simulink model "HIL_model_experiments1"  (R2013a)
settings: Solver=ode5  StartTime=0.0  StopTime=simulationTime  FixedStep=0.1  RelTol=1e-3
values from neighbouring files (symbols this model uses):
  Di = [50 0 ... (first row only)    [theProgram.m]
  Dist_spv_rfp = sqrt( ( shipL_d(1) - Rfp(1) )^2 + (shipL_d(2) - Rfp(2) )^2 )    [theProgram.m]
  Ds = [-X_u 0 0 ... (first row only)    [theProgram.m]
  K_M = [ 1 0 0 ... (first row only)    [theProgram.m]
  K_tow = 20    [theProgram.m]
  kappa = 2    [theProgram.m]
  Mi_a = iceMass*[1 0; 0 1]    [theProgram.m]
  Mi_rb = iceMass*[1 0; 0 1]    [theProgram.m]
  Ms_a = -[X_udot 0 0 ... (first row only)    [theProgram.m]
  Ms_rb = [shipMass 0 0 ... (first row only)    [theProgram.m]
  Ninstances = 50    [theProgram.m]
  overturnLimit = 4    [theProgram.m]
  Piceberg = [-4.5; -2.9]    [theProgram.m]
  Pship = [-3.5; -2.9; 0]    [theProgram.m]
  ruptureLimit = 3    [theProgram.m]
  saved_init = zeros(Ninstances,1)    [theProgram.m]
  sd_break = 0.075*T_break    (= 12)    [theProgram.m]
  sd_overturn = 0.075*T_overturn    (= 9.75)    [theProgram.m]
  sd_slip = 0.075*T_slip    (= 10.5)    [theProgram.m]
  simCase = 1    [theProgram.m]
  slippageLimit = 5    [theProgram.m]
  T_break = 160    [theProgram.m]
  T_overturn = 130    [theProgram.m]
  T_slip = 140    [theProgram.m]
  TowLineLength = 1.11    [theProgram.m]
  Vc = [cVelocity*cos(cAngle) ... (first row only)    [theProgram.m]
  vesselForces = [4; -1; 0]    [theProgram.m]
libraries: dspmtrx3 x1
settings Model: Creator=Andreas  LastModifiedBy=Andreas

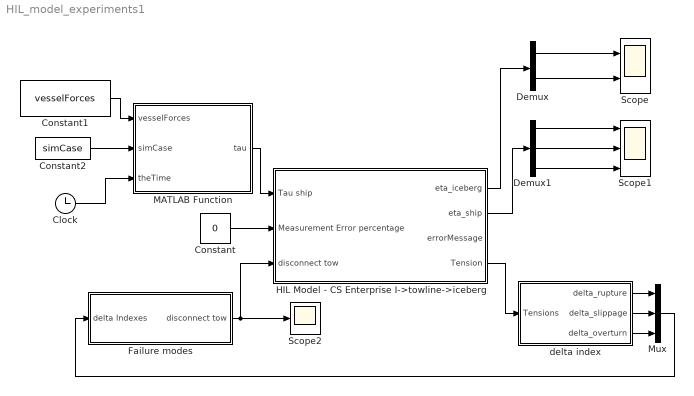
== system HIL_model_experiments1 ==
  Clock : Clock
  Constant : Constant  Value=0
  Constant1 : Constant  Value=vesselForces  VectorParams1D=off
  Constant2 : Constant  Value=simCase
  Demux : Demux  Outputs=2
  Demux1 : Demux  Outputs=3
  Failure modes : Subsystem
  HIL Model - CS Enterprise I->towline->iceberg : Subsystem  VariantControl=Variant1
  MATLAB Function : MATLAB Function  TreatAsAtomicUnit=on
  Mux : Mux  Inputs=3
  Scope : Scope  NumInputPorts=2
      settings: YMin=-5~-5  YMax=5~5  SaveName=ScopeData5
  Scope1 : Scope  NumInputPorts=3
      settings: YMin=-5~-5~-5  YMax=5~5~5  SaveName=ScopeData6
  Scope2 : Scope
      settings: SaveName=ScopeData7
  delta index : Subsystem
  wires:
  Constant/1 -> HIL Model - CS Enterprise I->towline->iceberg/2(Measurement Error percentage)
  HIL Model - CS Enterprise I->towline->iceberg/4(Tension) -> delta index/1(Tensions)
  Failure modes/1(disconnect tow) -> HIL Model - CS Enterprise I->towline->iceberg/3(disconnect tow), Scope2/1
  delta index/2(delta_slippage) -> Mux/2
  delta index/3(delta_overturn) -> Mux/3
  delta index/1(delta_rupture) -> Mux/1
  Mux/1 -> Failure modes/1(delta Indexes)
  HIL Model - CS Enterprise I->towline->iceberg/1(eta_iceberg) -> Demux/1
  Demux/2 -> Scope/2
  Demux/1 -> Scope/1
  HIL Model - CS Enterprise I->towline->iceberg/2(eta_ship) -> Demux1/1
  Demux1/2 -> Scope1/2
  Demux1/3 -> Scope1/3
  Demux1/1 -> Scope1/1
  MATLAB Function/1(tau) -> HIL Model - CS Enterprise I->towline->iceberg/1(Tau ship)
  Constant1/1 -> MATLAB Function/1(vesselForces)
  Constant2/1 -> MATLAB Function/2(simCase)
  Clock/1 -> MATLAB Function/3(theTime)

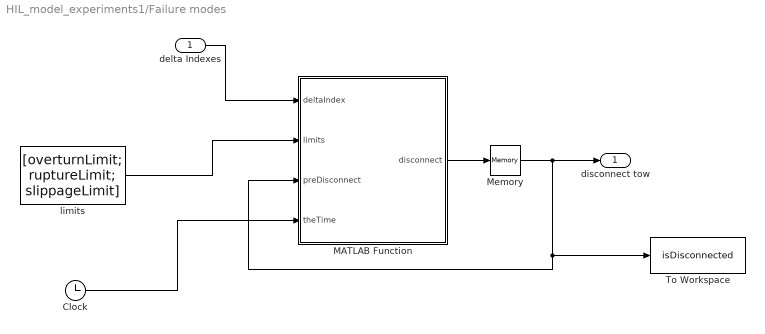
== system HIL_model_experiments1/Failure modes ==
  delta Indexes : Inport
  Clock : Clock
  MATLAB Function : MATLAB Function  TreatAsAtomicUnit=on
  Memory : Memory
  To Workspace : ToWorkspace  VariableName=isDisconnected  SampleTime=-1  SaveFormat=Timeseries
  limits : Constant  Value=[overturnLimit; ruptureLimit; slippageLimit]  VectorParams1D=off
  disconnect tow : Outport
  wires:
  limits/1 -> MATLAB Function/2(limits)
  delta Indexes/1 -> MATLAB Function/1(deltaIndex)
  Clock/1 -> MATLAB Function/4(theTime)
  MATLAB Function/1(disconnect) -> Memory/1
  Memory/1 -> MATLAB Function/3(preDisconnect), To Workspace/1, disconnect tow/1

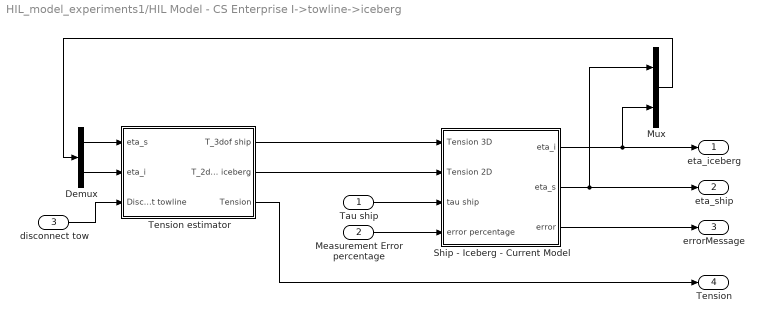
== system HIL_model_experiments1/HIL Model - CS Enterprise I->towline->iceberg ==
  Tau ship : Inport
  Measurement Error percentage : Inport  Port=2
  disconnect tow : Inport  Port=3
  Demux : Demux  Outputs=2
  Mux : Mux  Inputs=[3; 2]
  Ship - Iceberg - Current Model : Subsystem
  Tension estimator : Subsystem
  eta_iceberg : Outport
  eta_ship : Outport  Port=2
  errorMessage : Outport  Port=3
  Tension : Outport  Port=4
  wires:
  Tension estimator/2(T_2dof iceberg) -> Ship - Iceberg - Current Model/2(Tension 2D)
  Tension estimator/1(T_3dof ship) -> Ship - Iceberg - Current Model/1(Tension 3D)
  Measurement Error percentage/1 -> Ship - Iceberg - Current Model/4(error percentage)
  Demux/2 -> Tension estimator/2(eta_i)
  Ship - Iceberg - Current Model/1(eta_i) -> Mux/2, eta_iceberg/1
  Demux/1 -> Tension estimator/1(eta_s)
  Tau ship/1 -> Ship - Iceberg - Current Model/3(tau ship)
  Ship - Iceberg - Current Model/3(error) -> errorMessage/1
  Mux/1 -> Demux/1
  Ship - Iceberg - Current Model/2(eta_s) -> Mux/1, eta_ship/1
  Tension estimator/3(Tension) -> Tension/1
  disconnect tow/1 -> Tension estimator/3(Disconnect towline)

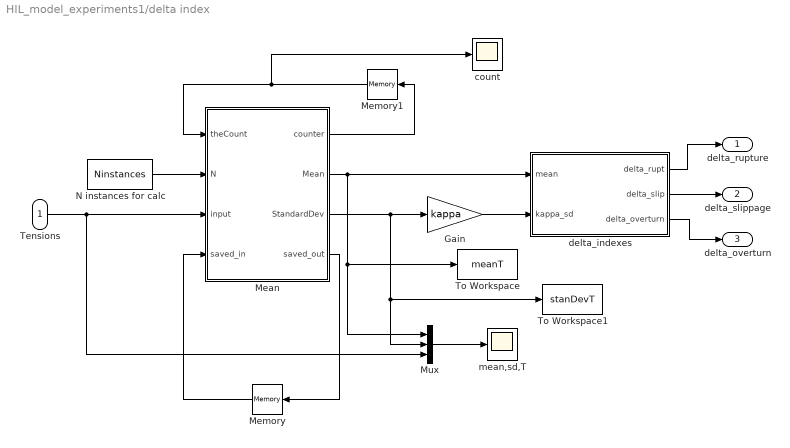
== system HIL_model_experiments1/delta index ==
  Tensions : Inport
  Gain : Gain  Gain=kappa
  Mean : MATLAB Function  TreatAsAtomicUnit=on
  Memory : Memory  X0=saved_init
  Memory1 : Memory  X0=1
  Mux : Mux  Inputs=3
  N instances for calc : Constant  Value=Ninstances
  To Workspace : ToWorkspace  VariableName=meanT  SampleTime=-1  SaveFormat=Timeseries
  To Workspace1 : ToWorkspace  VariableName=stanDevT  SampleTime=-1  SaveFormat=Timeseries
  count : Scope
  delta_indexes : Subsystem
  mean,sd,T : Scope
      settings: SaveName=ScopeData2
  delta_rupture : Outport
  delta_slippage : Outport  Port=2
  delta_overturn : Outport  Port=3
  wires:
  Mux/1 -> mean,sd,T/1
  Memory/1 -> Mean/4(saved_in)
  Memory1/1 -> Mean/1(theCount), count/1
  Mean/3(StandardDev) -> To Workspace1/1, Mux/2, Gain/1
  Mean/1(counter) -> Memory1/1
  N instances for calc/1 -> Mean/2(N)
  Mean/4(saved_out) -> Memory/1
  Mean/2(Mean) -> Mux/1, To Workspace/1, delta_indexes/1(mean)
  Tensions/1 -> Mux/3, Mean/3(input)
  Gain/1 -> delta_indexes/2(kappa_sd)
  delta_indexes/1(delta_rupt) -> delta_rupture/1
  delta_indexes/2(delta_slip) -> delta_slippage/1
  delta_indexes/3(delta_overturn) -> delta_overturn/1

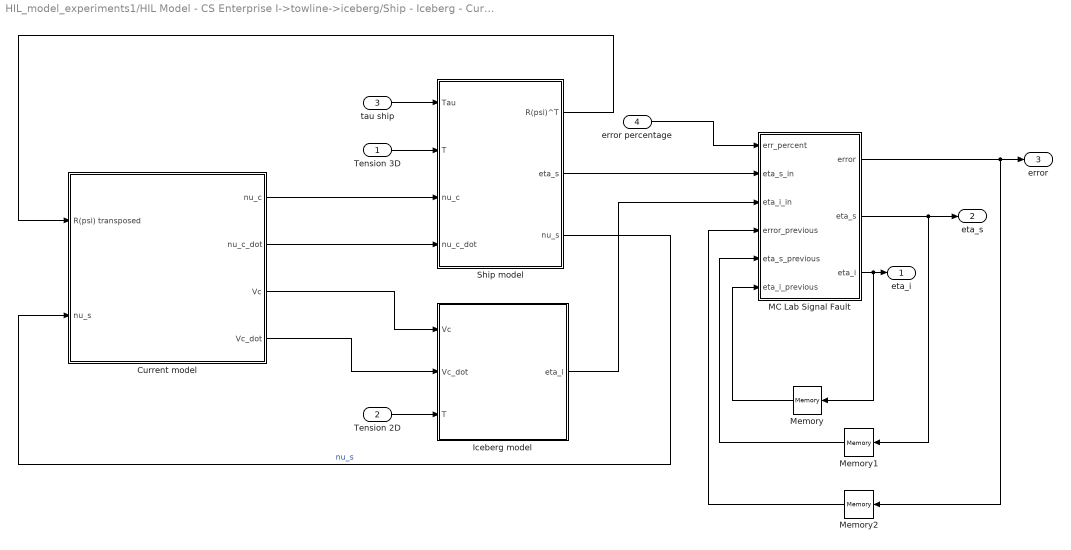
== system HIL_model_experiments1/HIL Model - CS Enterprise I->towline->iceberg/Ship - Iceberg - Current Model ==
  Tension 3D : Inport
  Tension 2D : Inport  Port=2
  tau ship : Inport  Port=3
  error percentage : Inport  Port=4
  Current model : Subsystem
  Iceberg model : Subsystem
  MC Lab Signal Fault : MATLAB Function  TreatAsAtomicUnit=on
  Memory : Memory  X0=[0; 0]
  Memory1 : Memory  X0=[0; 0; 0]
  Memory2 : Memory
  Ship model : Subsystem
  eta_i : Outport
  eta_s : Outport  Port=2
  error : Outport  Port=3
  wires:
  Memory2/1 -> MC Lab Signal Fault/4(error_previous)
  Memory1/1 -> MC Lab Signal Fault/5(eta_s_previous)
  Memory/1 -> MC Lab Signal Fault/6(eta_i_previous)
  MC Lab Signal Fault/1(error) -> error/1, Memory2/1
  MC Lab Signal Fault/3(eta_i) -> eta_i/1, Memory/1
  MC Lab Signal Fault/2(eta_s) -> eta_s/1, Memory1/1
  Iceberg model/1(eta_i) -> MC Lab Signal Fault/3(eta_i_in)
  Ship model/2(eta_s) -> MC Lab Signal Fault/2(eta_s_in)
  error percentage/1 -> MC Lab Signal Fault/1(err_percent)
  Ship model/3(nu_s) -> Current model/2(nu_s)  "nu_s"
  Ship model/1(R(psi)^T) -> Current model/1(R(psi) transposed)
  Tension 2D/1 -> Iceberg model/3(T)
  Current model/4(Vc_dot) -> Iceberg model/2(Vc_dot)
  Current model/3(Vc) -> Iceberg model/1(Vc)
  Current model/2(nu_c_dot) -> Ship model/4(nu_c_dot)
  Current model/1(nu_c) -> Ship model/3(nu_c)
  Tension 3D/1 -> Ship model/2(T)
  tau ship/1 -> Ship model/1(Tau)

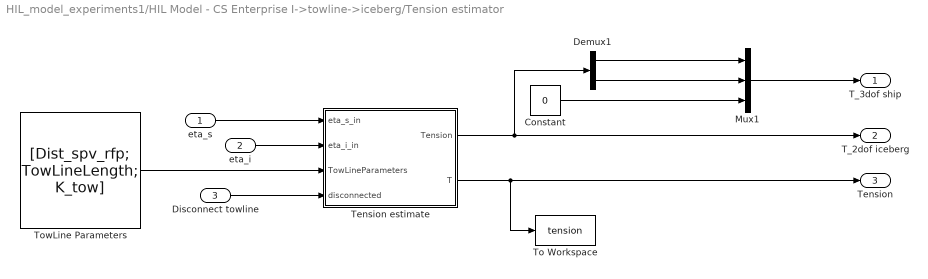
== system HIL_model_experiments1/HIL Model - CS Enterprise I->towline->iceberg/Tension estimator ==
  eta_s : Inport
  eta_i : Inport  Port=2
  Disconnect towline : Inport  Port=3
  Constant : Constant  Value=0
  Demux1 : Demux  Outputs=2
  Mux1 : Mux  Inputs=3
  Tension estimate : MATLAB Function  TreatAsAtomicUnit=on
  To Workspace : ToWorkspace  VariableName=tension  SampleTime=-1  SaveFormat=Timeseries
  TowLine Parameters : Constant  Value=[Dist_spv_rfp; TowLineLength; K_tow]  VectorParams1D=off
  T_3dof ship : Outport
  T_2dof iceberg : Outport  Port=2
  Tension : Outport  Port=3
  wires:
  Tension estimate/1(Tension) -> T_2dof iceberg/1, Demux1/1
  TowLine Parameters/1 -> Tension estimate/3(TowLineParameters)
  Constant/1 -> Mux1/3
  Demux1/2 -> Mux1/2
  Demux1/1 -> Mux1/1
  Mux1/1 -> T_3dof ship/1
  eta_s/1 -> Tension estimate/1(eta_s_in)
  eta_i/1 -> Tension estimate/2(eta_i_in)
  Tension estimate/2(T) -> To Workspace/1, Tension/1
  Disconnect towline/1 -> Tension estimate/4(disconnected)

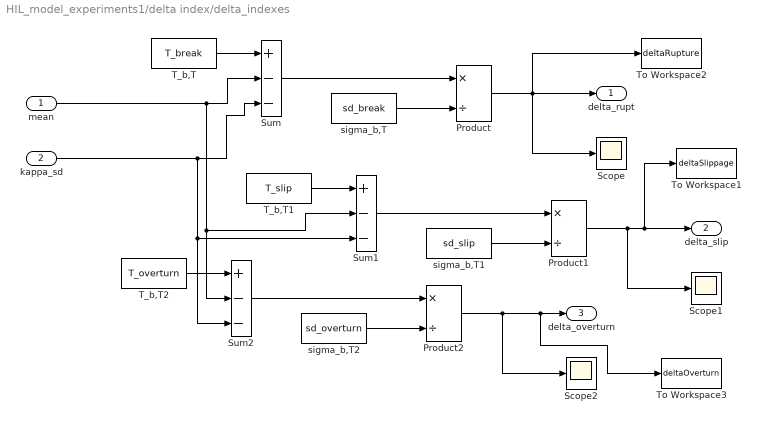
== system HIL_model_experiments1/delta index/delta_indexes ==
  mean : Inport
  kappa_sd : Inport  Port=2
  Product : Product  Inputs=*/
  Product1 : Product  Inputs=*/
  Product2 : Product  Inputs=*/
  Scope : Scope
  Scope1 : Scope
      settings: SaveName=ScopeData3
  Scope2 : Scope
      settings: SaveName=ScopeData4
  Sum : Sum  Inputs=+--
  Sum1 : Sum  Inputs=+--
  Sum2 : Sum  Inputs=+--
  T_b,T : Constant  Value=T_break
  T_b,T1 : Constant  Value=T_slip
  T_b,T2 : Constant  Value=T_overturn
  To Workspace1 : ToWorkspace  VariableName=deltaSlippage  SampleTime=-1  SaveFormat=Timeseries
  To Workspace2 : ToWorkspace  VariableName=deltaRupture  SampleTime=-1  SaveFormat=Timeseries
  To Workspace3 : ToWorkspace  VariableName=deltaOverturn  SampleTime=-1  SaveFormat=Timeseries
  sigma_b,T : Constant  Value=sd_break
  sigma_b,T1 : Constant  Value=sd_slip
  sigma_b,T2 : Constant  Value=sd_overturn
  delta_rupt : Outport
  delta_slip : Outport  Port=2
  delta_overturn : Outport  Port=3
  wires:
  Product/1 -> To Workspace2/1, delta_rupt/1, Scope/1
  kappa_sd/1 -> Sum2/3, Sum1/3, Sum/3
  sigma_b,T/1 -> Product/2
  Sum/1 -> Product/1
  T_b,T/1 -> Sum/1
  mean/1 -> Sum2/2, Sum1/2, Sum/2
  Product1/1 -> To Workspace1/1, delta_slip/1, Scope1/1
  sigma_b,T1/1 -> Product1/2
  Sum1/1 -> Product1/1
  T_b,T1/1 -> Sum1/1
  Product2/1 -> To Workspace3/1, delta_overturn/1, Scope2/1
  sigma_b,T2/1 -> Product2/2
  Sum2/1 -> Product2/1
  T_b,T2/1 -> Sum2/1

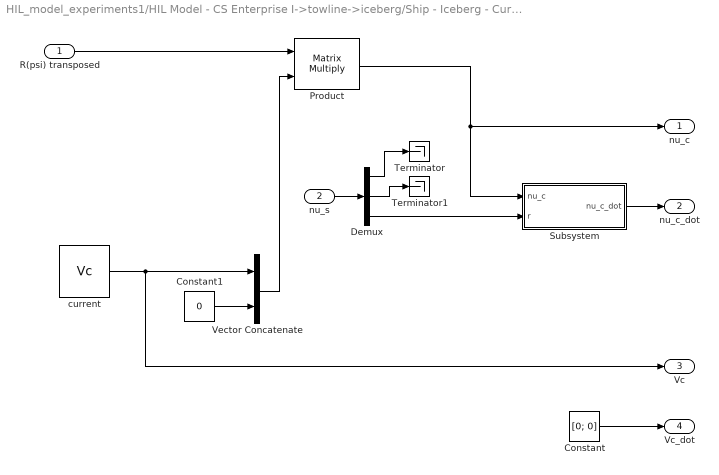
== system HIL_model_experiments1/HIL Model - CS Enterprise I->towline->iceberg/Ship - Iceberg - Current Model/Current model ==
  R(psi) transposed : Inport
  nu_s : Inport  Port=2
  Constant : Constant  Value=[0; 0]  VectorParams1D=off
  Constant1 : Constant  Value=0
  Demux : Demux  Outputs=3
  Product : Product  Multiplication=Matrix(*)
  Subsystem : Subsystem
  Terminator : Terminator
  Terminator1 : Terminator
  Vector Concatenate : Concatenate  Mode=Multidimensional array
  current : Constant  Value=Vc  VectorParams1D=off
  nu_c : Outport
  nu_c_dot : Outport  Port=2
  Vc : Outport  Port=3
  Vc_dot : Outport  Port=4
  wires:
  Vector Concatenate/1 -> Product/2
  Constant1/1 -> Vector Concatenate/2
  Constant/1 -> Vc_dot/1
  Subsystem/1(nu_c_dot) -> nu_c_dot/1
  Demux/3 -> Subsystem/2(r)
  Demux/2 -> Terminator1/1
  Demux/1 -> Terminator/1
  nu_s/1 -> Demux/1
  Product/1 -> nu_c/1, Subsystem/1(nu_c)
  R(psi) transposed/1 -> Product/1
  current/1 -> Vector Concatenate/1, Vc/1

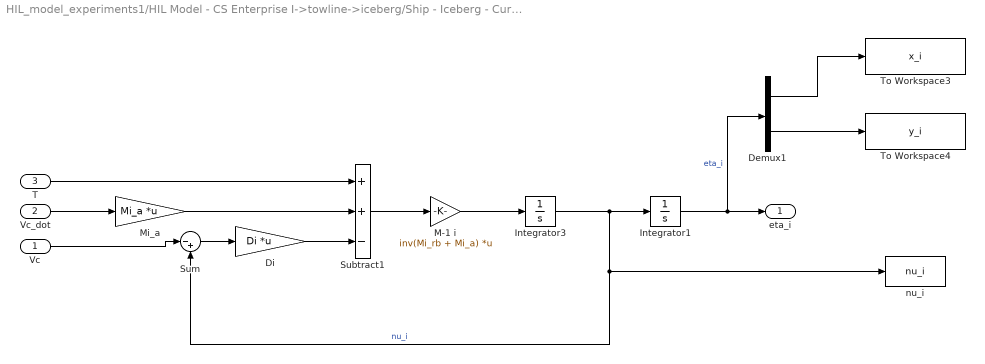
== system HIL_model_experiments1/HIL Model - CS Enterprise I->towline->iceberg/Ship - Iceberg - Current Model/Iceberg model ==
  Vc : Inport
  Vc_dot : Inport  Port=2
  T : Inport  Port=3
  Demux1 : Demux  Outputs=2
  Di : Gain  Gain=Di  Multiplication=Matrix(K*u) (u vector)
  Integrator1 : Integrator  InitialCondition=Piceberg
  Integrator3 : Integrator  InitialCondition=[0;0]
  M-1 i : Gain  Gain=inv(Mi_rb + Mi_a)  Multiplication=Matrix(K*u)
  Mi_a : Gain  Gain=Mi_a  Multiplication=Matrix(K*u) (u vector)
  Subtract1 : Sum  Inputs=++-
  Sum : Sum  Inputs=|-+
  To Workspace3 : ToWorkspace  VariableName=x_i  SampleTime=-1  SaveFormat=Timeseries
  To Workspace4 : ToWorkspace  VariableName=y_i  SampleTime=-1  SaveFormat=Timeseries
  nu_i : ToWorkspace  VariableName=nu_i  SampleTime=-1  SaveFormat=Timeseries
  eta_i : Outport
  wires:
  Demux1/2 -> To Workspace4/1
  Demux1/1 -> To Workspace3/1
  Di/1 -> Subtract1/3
  Sum/1 -> Di/1
  Vc/1 -> Sum/1
  Mi_a/1 -> Subtract1/2
  Vc_dot/1 -> Mi_a/1
  T/1 -> Subtract1/1
  Subtract1/1 -> M-1 i/1
  M-1 i/1 -> Integrator3/1
  Integrator1/1 -> eta_i/1, Demux1/1  "eta_i"
  Integrator3/1 -> Integrator1/1, nu_i/1, Sum/2  "nu_i"

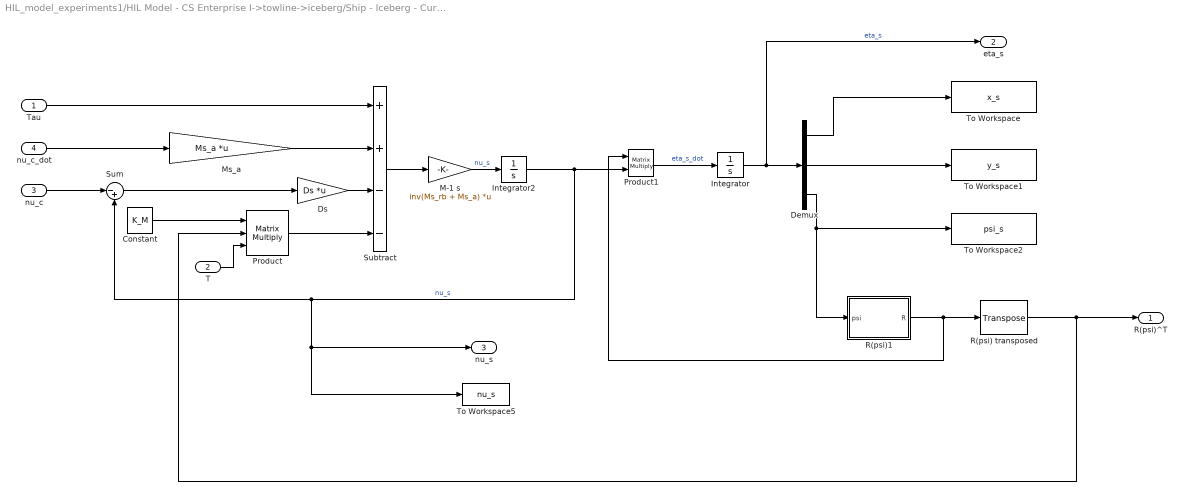
== system HIL_model_experiments1/HIL Model - CS Enterprise I->towline->iceberg/Ship - Iceberg - Current Model/Ship model ==
  Tau : Inport
  T : Inport  Port=2
  nu_c : Inport  Port=3
  nu_c_dot : Inport  Port=4
  Constant : Constant  Value=K_M  VectorParams1D=off
  Demux : Demux  Outputs=3
  Ds : Gain  Gain=Ds  Multiplication=Matrix(K*u) (u vector)
  Integrator : Integrator  InitialCondition=Pship
  Integrator2 : Integrator  InitialCondition=[0; 0; 0]
  M-1 s : Gain  Gain=inv(Ms_rb + Ms_a)  Multiplication=Matrix(K*u) (u vector)
  Ms_a : Gain  Gain=Ms_a  Multiplication=Matrix(K*u) (u vector)
  Product : Product  Inputs=***  Multiplication=Matrix(*)
  Product1 : Product  Multiplication=Matrix(*)
  R(psi) transposed : dspmtrx3/Transpose  Hermitian=off  overflowFlag=off
  R(psi)1 : MATLAB Function  TreatAsAtomicUnit=on
  Subtract : Sum  Inputs=++--
  Sum : Sum  Inputs=|-+
  To Workspace : ToWorkspace  VariableName=x_s  SampleTime=-1  SaveFormat=Timeseries
  To Workspace1 : ToWorkspace  VariableName=y_s  SampleTime=-1  SaveFormat=Timeseries
  To Workspace2 : ToWorkspace  VariableName=psi_s  SampleTime=-1  SaveFormat=Timeseries
  To Workspace5 : ToWorkspace  VariableName=nu_s  SampleTime=-1  SaveFormat=Timeseries
  R(psi)^T : Outport
  eta_s : Outport  Port=2
  nu_s : Outport  Port=3
  wires:
  Tau/1 -> Subtract/1
  R(psi) transposed/1 -> Product/2, R(psi)^T/1
  Demux/3 -> To Workspace2/1, R(psi)1/1(psi)
  Demux/2 -> To Workspace1/1
  Demux/1 -> To Workspace/1
  Product1/1 -> Integrator/1  "eta_s_dot"
  R(psi)1/1(R) -> Product1/1, R(psi) transposed/1
  Constant/1 -> Product/1
  Subtract/1 -> M-1 s/1
  M-1 s/1 -> Integrator2/1  "nu_s"
  Ds/1 -> Subtract/3
  Ms_a/1 -> Subtract/2
  Integrator/1 -> Demux/1, eta_s/1  "eta_s"
  T/1 -> Product/3
  nu_c/1 -> Sum/1
  Sum/1 -> Ds/1
  Integrator2/1 -> Product1/2, nu_s/1, To Workspace5/1, Sum/2  "nu_s"
  Product/1 -> Subtract/4
  nu_c_dot/1 -> Ms_a/1

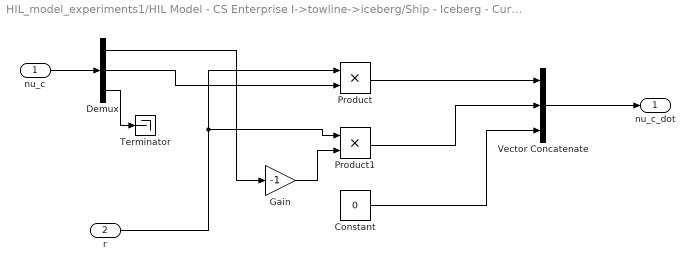
== system HIL_model_experiments1/HIL Model - CS Enterprise I->towline->iceberg/Ship - Iceberg - Current Model/Current model/Subsystem ==
  nu_c : Inport
  r : Inport  Port=2
  Constant : Constant  Value=0
  Demux : Demux  Outputs=3
  Gain : Gain  Gain=-1
  Product : Product
  Product1 : Product
  Terminator : Terminator
  Vector Concatenate : Concatenate  NumInputs=3  Mode=Multidimensional array
  nu_c_dot : Outport
  wires:
  Gain/1 -> Product1/2
  Demux/1 -> Gain/1
  Demux/2 -> Product/2
  r/1 -> Product/1, Product1/1
  Constant/1 -> Vector Concatenate/3
  Product1/1 -> Vector Concatenate/2
  Product/1 -> Vector Concatenate/1
  Vector Concatenate/1 -> nu_c_dot/1
  Demux/3 -> Terminator/1
  nu_c/1 -> Demux/1

== matlab function HIL_model_experiments1/HIL Model - CS Enterprise I->towline->iceberg/Ship - Iceberg - Current Model/MC Lab Signal Fault ==
  data: error output; err_percent input; eta_s output; eta_s_in input; eta_i_in input; error_previous input; eta_s_previous input; eta_i_previous input; eta_i output
function [error, eta_s, eta_i] = fcn(err_percent, eta_s_in, eta_i_in, error_previous, eta_s_previous, eta_i_previous)
%#codegen


% Random number generator 0-100
num = 100*rand;

if error_previous == 1
    err_percent = 95;
end

% Check if the num is below the error percentage
if num < err_percent
    error = 1;
    eta_s = eta_s_previous;
    eta_i = eta_i_previous;
else
    error = 0;
    eta_s = eta_s_in;
    eta_i = eta_i_in;
end

== matlab function HIL_model_experiments1/HIL Model - CS Enterprise I->towline->iceberg/Ship - Iceberg - Current Model/Ship model/R(psi)1 ==
  data: psi input; R output
function R = fcn(psi)

c = cos(psi);
s = sin(psi);

R = [c -s 0;
     s c 0;
     0 0 1];

== matlab function HIL_model_experiments1/delta index/Mean ==
  data: counter output; theCount input; N input; Mean output; StandardDev output; input input; saved_in input; saved_out output
function [counter, Mean, StandardDev, saved_out] = fcn(theCount, N, input, saved_in)
%#codegen

meanSum = 0;
varSum = 0;

N = round(N);

startval = 2;
Ndiv = N;
if theCount < N
    startval = N + 1 - theCount;
    Ndiv = theCount;
end

% Bump all saved instances up
saved_out = saved_in;
for i=startval:N
    saved_out(i-1) = saved_in(i);
    meanSum = meanSum + saved_in(i);
end
saved_out(N) = input;
meanSum = meanSum + input;

Mean = (1/Ndiv)*meanSum;


% Calculate variance sum
for i=startval-1:N
    varSum = (saved_out(i) - Mean)^2;
end

variance = (1/Ndiv)*varSum;
StandardDev = sqrt(variance);

counter = theCount + 1;

== matlab function HIL_model_experiments1/HIL Model - CS Enterprise I->towline->iceberg/Tension estimator/Tension estimate ==
  data: eta_s_in input; Tension output; eta_i_in input; TowLineParameters input; T output; disconnected input
function [Tension, T] = fcn(eta_s_in,eta_i_in,TowLineParameters, disconnected)
%#codegen

if length(eta_s_in) > 1
    eta_s = eta_s_in;
else
    eta_s = [0; 0; 0];
end
if length(eta_i_in) > 1
    eta_i = eta_i_in;
else
    eta_i = [0; 0];
end

if disconnected == 0

    d = TowLineParameters(1);
    Tlength = TowLineParameters(2);
    K_tow = TowLineParameters(3);

    x_s = eta_s(1);
    y_s = eta_s(2);
    psi_s = eta_s(3);

    x_i = eta_i(1);
    y_i = eta_i(2);

    % Find rope fastening position in cartesian
    x_r = x_s - d*cos(psi_s);
    y_r = y_s - d*sin(psi_s);

    % Find towline fastening distance and angle
    dist = sqrt( (x_r - x_i)^2 + (y_r - y_i)^2 );
    angle = atan2(y_r-y_i, x_r-x_i);

    % Check if longer than rope length, because only rope stretching tension gives force
    T = 0;
    if dist >= Tlength

        deltaL = dist-Tlength;
        T = K_tow*deltaL;

    end

    % Make Xtow and Ytow
    Xtow = T*cos(angle);
    Ytow = T*sin(angle);

    Tension = [Xtow; Ytow];

else
    
    T = 0;
    Tension = [0; 0];
    
end

== matlab function HIL_model_experiments1/Failure modes/MATLAB Function ==
  data: deltaIndex input; disconnect output; limits input; preDisconnect input; theTime input
function disconnect = fcn(deltaIndex, limits, preDisconnect, theTime)
%#codegen

disconnect = preDisconnect;

if preDisconnect == 0 && theTime > 0

    deltaOverturn = deltaIndex(3);
    deltaRupture = deltaIndex(1);
    deltaSlippage = deltaIndex(2);
    
    overturn = limits(1);
    rupture = limits(2);
    slippage = limits(3);
    
    if deltaOverturn < overturn

        theTime
        disp('Iceberg has overturned, towline is disconnected.');
        disconnect = 1;
        
    elseif deltaRupture < rupture
        
        theTime
        disp('Towline has ruptured, and is disconnected.');
        disconnect = 1;
        
    elseif deltaSlippage < slippage
        
        theTime
        disp('Towline has slipped, and is disconnected.');
        disconnect = 1;
        
    end
    
end

== matlab function HIL_model_experiments1/MATLAB Function ==
  data: vesselForces input; tau output; simCase input; theTime input
function tau = fcn(vesselForces, simCase, theTime)

tau = vesselForces;
if simCase == 4 % Linear, rising force
    
    tau = vesselForces * theTime;
    
end
